simulink model "RC_Circuit"  (R2020a)
settings: Solver=VariableStepAuto  StartTime=0.0  StopTime=10.0  RelTol=1e-3
undefined symbols (not defined in the file): C, R
settings Model: Creator=NIKITA  LastModifiedBy=NIKITA

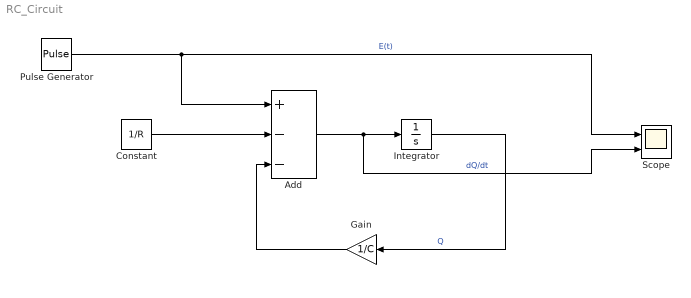
== system RC_Circuit ==
  Add : Sum  Inputs=+--
  Constant : Constant  Value=1/R
  Gain : Gain  Gain=1/C
  Integrator : Integrator
  Pulse Generator : DiscretePulseGenerator  PulseType=Time based  Period=10  PulseWidth=5
  Scope : Scope  NumInputPorts=2
  wires:
  Add/1 -> Scope/2, Integrator/1  "dQ/dt"
  Integrator/1 -> Gain/1  "Q"
  Pulse Generator/1 -> Scope/1, Add/1  "E(t)"
  Gain/1 -> Add/3
  Constant/1 -> Add/2
